simulink model "State_estimation"  (R2018b)
settings: Solver=VariableStepAuto  StartTime=0.0  StopTime=Time  RelTol=1e-3
values from neighbouring files (symbols this model uses):
  a0 = Wv^3    (= 10635152.9013)    [Cogging_ANAL.m]
  a1 = 3*Wv^2    (= 145083.184696)    [Cogging_ANAL.m]
  a2 = 3*Wv    (= 659.734457254)    [Cogging_ANAL.m]
  ts = 0.001    [Cogging_ANAL.m]
settings Model: Creator=Dave Vogel  LastModifiedBy=Dave Vogel
settings DebuggingCC: LibraryContextMissingDiagnostic=none
settings SFSimCC: SimUseLocalCustomCode=off
settings RTWCC: RTWUseLocalCustomCode=off

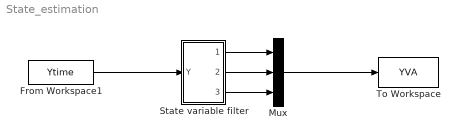
== system State_estimation ==
  From Workspace1 : FromWorkspace  VariableName=Ytime  SampleTime=ts  Interpolate=off  OutputAfterFinalValue=Setting to zero
  Mux : Mux  Inputs=3
  State variable filter : Subsystem
  To Workspace : ToWorkspace  VariableName=YVA  SaveFormat=Timeseries  SampleTime=ts
  wires:
  From Workspace1/1 -> State variable filter/1(Y)
  State variable filter/1(yest) -> Mux/1
  State variable filter/2(dyest) -> Mux/2
  State variable filter/3(ddyest) -> Mux/3
  Mux/1 -> To Workspace/1

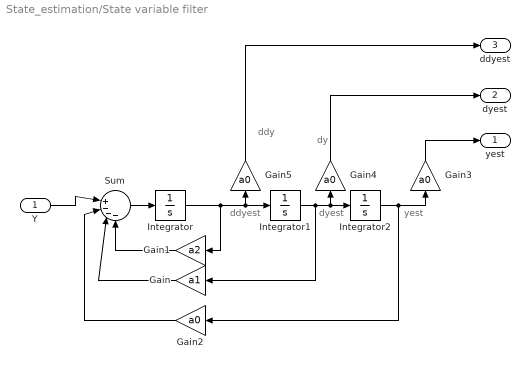
== system State_estimation/State variable filter ==
  note: dy
  note: ddy
  note: ddyest
  note: dyest
  note: yest
  Y : Inport
  Gain : Gain  Gain=a1
  Gain1 : Gain  Gain=a2
  Gain{2..5} (4 alike) : Gain  Gain=a0
  Integrator : Integrator
  Integrator1 : Integrator
  Integrator2 : Integrator
  Sum : Sum  Inputs=||+---
  yest : Outport  PortDimensions=1
  dyest : Outport  Port=2  PortDimensions=1
  ddyest : Outport  Port=3  PortDimensions=1
  wires:
  Integrator/1 -> Integrator1/1, Gain5/1, Gain1/1
  Integrator1/1 -> Gain/1, Integrator2/1, Gain4/1
  Sum/1 -> Integrator/1
  Gain/1 -> Sum/3
  Gain3/1 -> yest/1
  Integrator2/1 -> Gain3/1, Gain2/1
  Gain2/1 -> Sum/2
  Gain1/1 -> Sum/4
  Y/1 -> Sum/1
  Gain4/1 -> dyest/1
  Gain5/1 -> ddyest/1
